simulink model "hmiTestDualMyo"  (R2017a)
settings: Solver=FixedStepAuto  StartTime=0.0  StopTime=inf  RelTol=1e-3
libraries: vrlib x3, myo_lib x3, sldrtlib x1
settings Model: Creator=ricardog  LastModifiedBy=ricardog
settings SolverCC: AutoInsertRateTranBlk=on

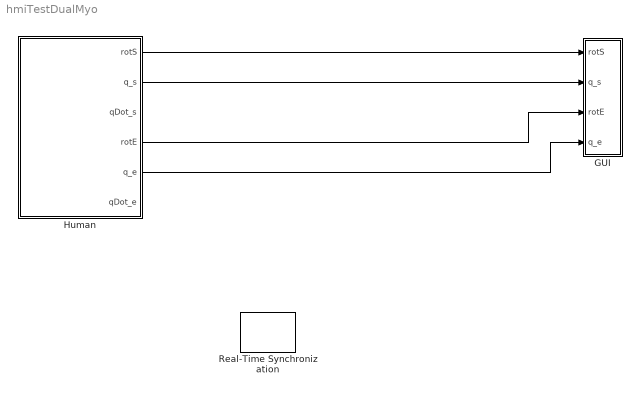
== system hmiTestDualMyo ==
  GUI : Subsystem
  Human : Subsystem
  Real-Time Synchronization : sldrtlib/Real-Time Synchronization  SampleTime=0.01  MaxMissedTicks=50  ShowMissedTicks=off  YieldWhenWaiting=off
  wires:
  Human/4(rotE) -> GUI/3(rotE)
  Human/5(q_e) -> GUI/4(q_e)
  Human/1(rotS) -> GUI/1(rotS)
  Human/2(q_s) -> GUI/2(q_s)

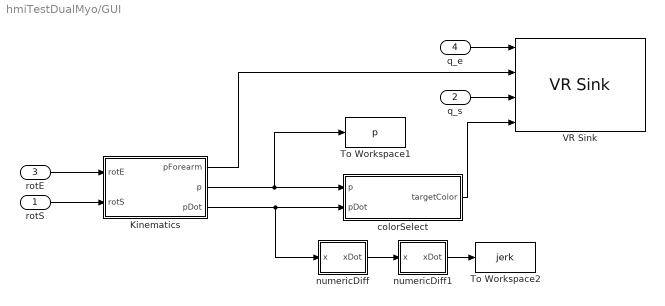
== system hmiTestDualMyo/GUI ==
  rotS : Inport
  q_s : Inport  Port=2
  rotE : Inport  Port=3
  q_e : Inport  Port=4
  Kinematics : Subsystem
  To Workspace1 : ToWorkspace  VariableName=p  SampleTime=-1
  To Workspace2 : ToWorkspace  VariableName=jerk  SampleTime=-1
  VR Sink : vrlib/VR Sink  InstantiateOnLoad=on  SampleTime=0.1  ViewEnable=on  RemoteChange=off  RemoteView=off  FieldsWritten=Forearm.rotation.4.1.1.double#Forearm.translation.3.1.1.double#UpperArm.rotation.4.1.1.double#EndTarget_material.diffuseColor.3.1.1.double  WorldFileName=C:\Users\ricardog\Documents\Workspace\HRSC_FW\GUI\armTargetsGUI.wrl  AutoView=on  VideoDimensions=[]  AllowVariableSize=off  FigureProperties="{'Position', 'Name', 'Viewpoint', 'CameraBound', 'CameraDirection', 'CameraPosition', 'CameraUpVector', 'ZoomFactor', 'Antialiasing', 'Headlight', 'Lighting', 'NavPanel', 'Sound', 'StatusBar', 'Stereo3D', 'Stereo3DCameraOffset', 'Stereo3DHIT', 'ToolBar', 'Textures', 'Transparency', 'Triad', 'Wireframe', 'NavZones', 'NavMode', 'NavSpeed', 'CaptureFileFormat', 'CaptureFileName', 'Record2DCompressMethod', 'Record2DCompressQuality', 'Record2D', 'Record2DFileName', 'Record2DFPS'; [7.5700000000000000e+02   1.3100000000000000e+02   7.6480000000000018e+02   5.7960000000000002e+02], '', 'FPV', 'on', [0.0000000000000000e+00   0.0000000000000000e+00  -1.0000000000000000e+00], [0.0000000000000000e+00   0.0000000000000000e+00   0.0000000000000000e+00], [0.0000000000000000e+00   1.0000000000000000e+00   0.0000000000000000e+00], [1.0000000000000000e+00], 'on', 'on', 'on', 'halfbar', 'on', 'on', 'off', [1.0000000149011612e-01], [0.0000000000000000e+00], 'on', 'on', 'on', 'none', 'off', 'off', 'examine', 'normal', 'tif', '%f_anim_%n.tif', 'auto', [7.5000000000000000e+01], 'off', '%f_anim_%n.avi', 'auto'}"
      settings: SourceProductBaseCode=VR
  colorSelect : MATLAB Function  TreatAsAtomicUnit=on
  numericDiff : Subsystem
  numericDiff1 : Subsystem
  wires:
  Kinematics/1(pForearm) -> VR Sink/2
  numericDiff/1(xDot) -> numericDiff1/1(x)
  Kinematics/3(pDot) -> numericDiff/1(x), colorSelect/2(pDot)
  Kinematics/2(p) -> To Workspace1/1, colorSelect/1(p)
  numericDiff1/1(xDot) -> To Workspace2/1
  q_e/1 -> VR Sink/1
  rotS/1 -> Kinematics/2(rotS)
  q_s/1 -> VR Sink/3
  rotE/1 -> Kinematics/1(rotE)
  colorSelect/1(targetColor) -> VR Sink/4

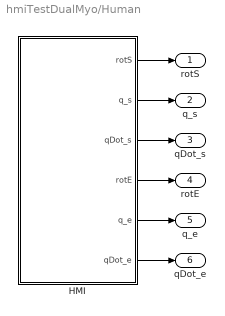
== system hmiTestDualMyo/Human ==
  HMI : Subsystem
  rotS : Outport
  q_s : Outport  Port=2
  qDot_s : Outport  Port=3
  rotE : Outport  Port=4
  q_e : Outport  Port=5
  qDot_e : Outport  Port=6
  wires:
  HMI/1(rotS) -> rotS/1
  HMI/2(q_s) -> q_s/1
  HMI/3(qDot_s) -> qDot_s/1
  HMI/4(rotE) -> rotE/1
  HMI/5(q_e) -> q_e/1
  HMI/6(qDot_e) -> qDot_e/1

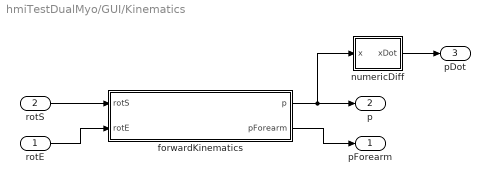
== system hmiTestDualMyo/GUI/Kinematics ==
  rotE : Inport
  rotS : Inport  Port=2
  forwardKinematics : MATLAB Function  TreatAsAtomicUnit=on
  numericDiff : Subsystem
  pForearm : Outport
  p : Outport  Port=2
  pDot : Outport  Port=3
  wires:
  forwardKinematics/1(p) -> numericDiff/1(x), p/1
  forwardKinematics/2(pForearm) -> pForearm/1
  rotS/1 -> forwardKinematics/1(rotS)
  rotE/1 -> forwardKinematics/2(rotE)
  numericDiff/1(xDot) -> pDot/1

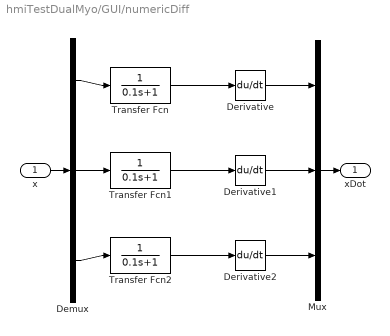
== system hmiTestDualMyo/GUI/numericDiff ==
  x : Inport
  Demux : Demux  Outputs=3
  Derivative : Derivative
  Derivative1 : Derivative
  Derivative2 : Derivative
  Mux : Mux  Inputs=3
  Transfer Fcn : TransferFcn  Denominator=[0.1 1]
  Transfer Fcn1 : TransferFcn  Denominator=[0.1 1]
  Transfer Fcn2 : TransferFcn  Denominator=[0.1 1]
  xDot : Outport
  wires:
  Mux/1 -> xDot/1
  Derivative1/1 -> Mux/2
  x/1 -> Demux/1
  Demux/3 -> Transfer Fcn2/1
  Derivative2/1 -> Mux/3
  Transfer Fcn/1 -> Derivative/1
  Demux/1 -> Transfer Fcn/1
  Derivative/1 -> Mux/1
  Transfer Fcn2/1 -> Derivative2/1
  Transfer Fcn1/1 -> Derivative1/1
  Demux/2 -> Transfer Fcn1/1

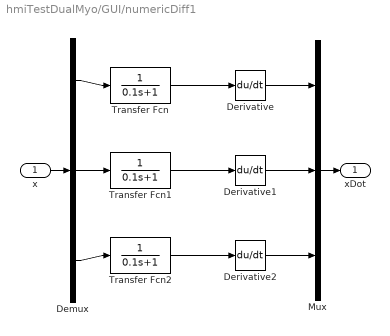
== system hmiTestDualMyo/GUI/numericDiff1 ==
  x : Inport
  Demux : Demux  Outputs=3
  Derivative : Derivative
  Derivative1 : Derivative
  Derivative2 : Derivative
  Mux : Mux  Inputs=3
  Transfer Fcn : TransferFcn  Denominator=[0.1 1]
  Transfer Fcn1 : TransferFcn  Denominator=[0.1 1]
  Transfer Fcn2 : TransferFcn  Denominator=[0.1 1]
  xDot : Outport
  wires:
  Mux/1 -> xDot/1
  Derivative1/1 -> Mux/2
  x/1 -> Demux/1
  Demux/3 -> Transfer Fcn2/1
  Derivative2/1 -> Mux/3
  Transfer Fcn/1 -> Derivative/1
  Demux/1 -> Transfer Fcn/1
  Derivative/1 -> Mux/1
  Transfer Fcn2/1 -> Derivative2/1
  Transfer Fcn1/1 -> Derivative1/1
  Demux/2 -> Transfer Fcn1/1

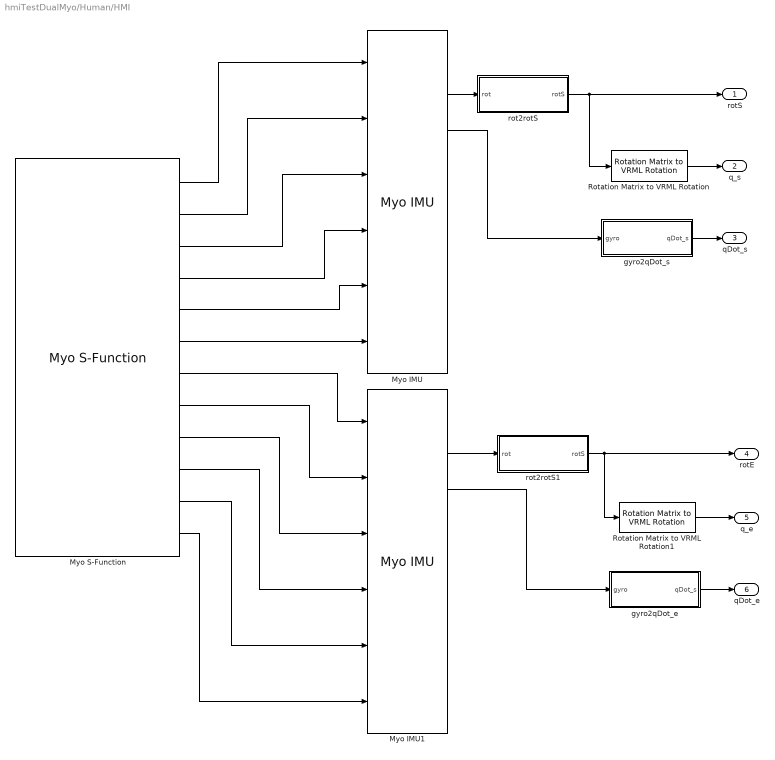
== system hmiTestDualMyo/Human/HMI ==
  Myo IMU : myo_lib/Myo IMU
  Myo IMU1 : myo_lib/Myo IMU
  Myo S-Function : myo_lib/Myo S-Function  emgEnabled=0  countMyos=2
  Rotation Matrix to VRML Rotation : vrlib/Utilities/Rotation Matrix to VRML Rotation  maxzero=1e-12
      settings: SourceProductName=Simulink 3D Animation  SourceProductBaseCode=VR
  Rotation Matrix to VRML Rotation1 : vrlib/Utilities/Rotation Matrix to VRML Rotation  maxzero=1e-12
      settings: SourceProductName=Simulink 3D Animation  SourceProductBaseCode=VR
  gyro2qDot_e : MATLAB Function  TreatAsAtomicUnit=on
  gyro2qDot_s : MATLAB Function  TreatAsAtomicUnit=on
  rot2rotS : MATLAB Function  TreatAsAtomicUnit=on
  rot2rotS1 : MATLAB Function  TreatAsAtomicUnit=on
  rotS : Outport
  q_s : Outport  Port=2
  qDot_s : Outport  Port=3
  rotE : Outport  Port=4
  q_e : Outport  Port=5
  qDot_e : Outport  Port=6
  wires:
  Myo S-Function/3 -> Myo IMU/3
  Myo S-Function/4 -> Myo IMU/4
  Myo S-Function/5 -> Myo IMU/5
  Myo S-Function/2 -> Myo IMU/2
  Myo S-Function/1 -> Myo IMU/1
  Myo S-Function/6 -> Myo IMU/6
  Myo S-Function/7 -> Myo IMU1/1
  Myo S-Function/8 -> Myo IMU1/2
  Myo S-Function/9 -> Myo IMU1/3
  Myo S-Function/10 -> Myo IMU1/4
  Myo S-Function/11 -> Myo IMU1/5
  Myo S-Function/12 -> Myo IMU1/6
  Myo IMU/2 -> rot2rotS/1(rot)
  rot2rotS/1(rotS) -> rotS/1, Rotation Matrix to VRML Rotation/1
  Rotation Matrix to VRML Rotation/1 -> q_s/1
  Myo IMU/3 -> gyro2qDot_s/1(gyro)
  Myo IMU1/2 -> rot2rotS1/1(rot)
  gyro2qDot_s/1(qDot_s) -> qDot_s/1
  rot2rotS1/1(rotS) -> Rotation Matrix to VRML Rotation1/1, rotE/1
  Rotation Matrix to VRML Rotation1/1 -> q_e/1
  Myo IMU1/3 -> gyro2qDot_e/1(gyro)
  gyro2qDot_e/1(qDot_s) -> qDot_e/1

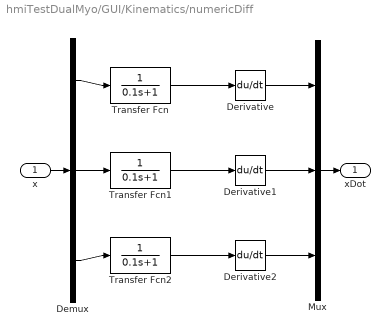
== system hmiTestDualMyo/GUI/Kinematics/numericDiff ==
  x : Inport
  Demux : Demux  Outputs=3
  Derivative : Derivative
  Derivative1 : Derivative
  Derivative2 : Derivative
  Mux : Mux  Inputs=3
  Transfer Fcn : TransferFcn  Denominator=[0.1 1]
  Transfer Fcn1 : TransferFcn  Denominator=[0.1 1]
  Transfer Fcn2 : TransferFcn  Denominator=[0.1 1]
  xDot : Outport
  wires:
  Mux/1 -> xDot/1
  Derivative1/1 -> Mux/2
  x/1 -> Demux/1
  Demux/3 -> Transfer Fcn2/1
  Derivative2/1 -> Mux/3
  Transfer Fcn/1 -> Derivative/1
  Demux/1 -> Transfer Fcn/1
  Derivative/1 -> Mux/1
  Transfer Fcn2/1 -> Derivative2/1
  Transfer Fcn1/1 -> Derivative1/1
  Demux/2 -> Transfer Fcn1/1

== matlab function hmiTestDualMyo/GUI/Kinematics/forwardKinematics ==
  data: rotS input; p output; rotE input; pForearm output
%
%
function [p,pForearm] = forwardKinematics(rotS,rotE)
% Get arm length
lA = get(armDynamics,'lA');
lF = get(armDynamics,'lF');
% Create distance vectors in local frame
rOA = [0;-lA;0];
rAF = [0;-lF;0];
rAGF = [0;-lF/2;0];
pOA = rotS*rOA;
% Hand position
p = pOA+rotE*rAF;
% Forearm centre of mass position (middle)
pForearm = pOA+rotE*rAGF;

== matlab function hmiTestDualMyo/GUI/colorSelect ==
  data: p input; targetColor output; pDot input
function targetColor = colorSelect(p,pDot)
p_f = [0.5969;-0.0670;-0.2];   % Desired end position
pNorm = norm(p-p_f);
pDotNorm = norm(pDot);
if(pNorm<0.03 && pDotNorm<0.05)
    R = 0;
    G = 1;
    B = 0;
else
    R = 0;
    G = 0;
    B = 1;
end
targetColor = [R;G;B];

== matlab function hmiTestDualMyo/Human/HMI/gyro2qDot_s ==
  data: gyro input; qDot_s output
% rot2rotS Converts fixed sensor frame sensor rotation matrix to VRML fixed
% frame.
% @in gyro gyroscope angular velocity vector.
% @out qDot_s shoulder angular velocity vector.
%
% Change log:
% Date        |   Comment           |     Owner
%-------------------------------------------------------
% 06/09/2017  | Creation            |     ricardog
% dd/mm/yyyy  | xxxxxxxxxxxxxxxx    |     xxxxxxxx
%
function qDot_s = gyro2qDot_s(gyro)
qDot_s = [1,-1,1].*deg2rad([gyro(3),gyro(2),gyro(1)]);

== matlab function hmiTestDualMyo/Human/HMI/rot2rotS ==
  data: rot input; rotS output
% rot2rotS Converts fixed sensor frame sensor rotation matrix to VRML fixed
% frame.
% @in rot fixed sensor frame sensor rotation matrix.
% @out rotS VRML fixed frame shoulder rotation matrix.
%
% Change log:
% Date        |   Comment           |     Owner
%-------------------------------------------------------
% 06/09/2017  | Creation            |     ricardog
% dd/mm/yyyy  | xxxxxxxxxxxxxxxx    |     xxxxxxxx
%
function rotS = rot2rotS(rot)
% Fixed sensor frame -90deg x rotation, fixed sensor frame rotation
% converts to VRML fixed frame. VRML fixed frame 90deg z rotation converts
% to shoulder zero frame.
rotS = rotx(-90)*rot*rotz(90)*roty(-90);

== matlab function hmiTestDualMyo/Human/HMI/rot2rotS1 ==
  data: rot input; rotS output
% rot2rotS Converts fixed sensor frame sensor rotation matrix to VRML fixed
% frame.
% @in rot fixed sensor frame sensor rotation matrix.
% @out rotS VRML fixed frame shoulder rotation matrix.
%
% Change log:
% Date        |   Comment           |     Owner
%-------------------------------------------------------
% 06/09/2017  | Creation            |     ricardog
% dd/mm/yyyy  | xxxxxxxxxxxxxxxx    |     xxxxxxxx
%
function rotS = rot2rotS(rot)
% Fixed sensor frame -90deg x rotation, fixed sensor frame rotation
% converts to VRML fixed frame. VRML fixed frame 90deg z rotation converts
% to shoulder zero frame.
rotS = rotx(-90)*rot*rotz(90)*roty(-90);

== matlab function hmiTestDualMyo/Human/HMI/gyro2qDot_e ==
  data: gyro input; qDot_s output
% rot2rotS Converts fixed sensor frame sensor rotation matrix to VRML fixed
% frame.
% @in gyro gyroscope angular velocity vector.
% @out qDot_s shoulder angular velocity vector.
%
% Change log:
% Date        |   Comment           |     Owner
%-------------------------------------------------------
% 06/09/2017  | Creation            |     ricardog
% dd/mm/yyyy  | xxxxxxxxxxxxxxxx    |     xxxxxxxx
%
function qDot_s = gyro2qDot_s(gyro)
qDot_s = [1,-1,1].*deg2rad([gyro(3),gyro(2),gyro(1)]);
